simulink model "VH_fb_scheme"  (Simulink 5.0)
settings: Solver=ode45  StartTime=0.0  StopTime=10.0  RelTol=1e-3
settings Model: Creator=andrisan  LastModifiedBy=andrisan  ExtModeAutoUpdateStatusClock=off

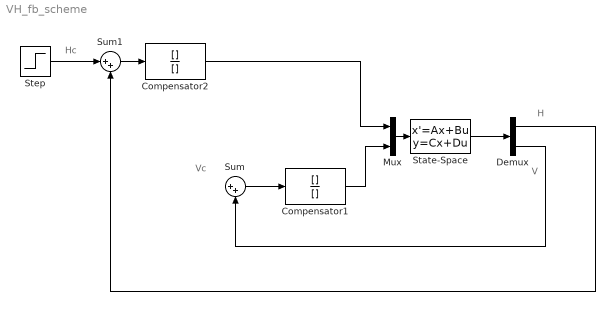
== system VH_fb_scheme ==
  note: Vc
  note: V
  note: H
  note: Hc
  Compensator1 : TransferFcn  Numerator=[]  Denominator=[]
  Compensator2 : TransferFcn  Numerator=[]  Denominator=[]
  Demux : Demux  Outputs=2
  Mux : Mux  Inputs=2
  State-Space : StateSpace
  Step : Step  SampleTime=0
  Sum : Sum  Inputs=|++  SaturateOnIntegerOverflow=on
  Sum1 : Sum  Inputs=|++  SaturateOnIntegerOverflow=on
  wires:
  Sum/1 -> Compensator1/1
  ? -> Sum/1
  State-Space/1 -> Demux/1
  Demux/2 -> Sum/2
  Sum1/1 -> Compensator2/1
  Mux/1 -> State-Space/1
  Compensator1/1 -> Mux/2
  Demux/1 -> Sum1/2
  Compensator2/1 -> Mux/1
  Step/1 -> Sum1/1
